simulink model "FormationControl"  (R2021b)
settings: Solver=VariableStepAuto  StartTime=0.0  StopTime=t_sim2  RelTol=1e-3
undefined symbols (not defined in the file or in its folder): d, form
libraries: instrumentlib x1
settings Model: PacingRate=0.100000  Creator=Cinthy  LastModifiedBy=Cinthy

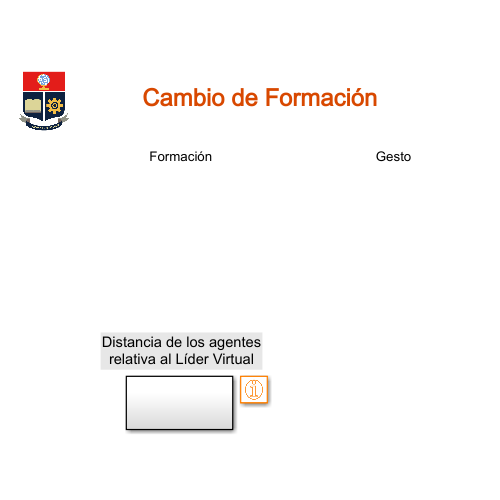
[thumbnail: Simulink's stored preview of the top-level diagram]
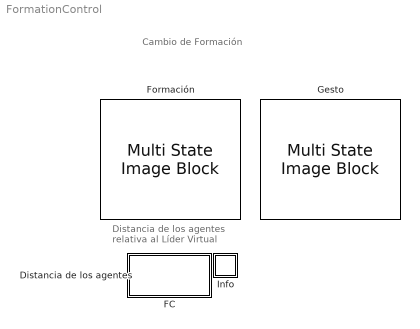
== system FormationControl ==
  note: Distancia de los agentes
      | relativa al Líder Virtual
  note: Cambio de Formación
  Distancia de los agentes : DisplayBlock  LabelPosition=Hide  Format=short  Transparency=1
  FC : Subsystem
  Formación : MultiStateImageBlock  LabelPosition=Hide
  Gesto : MultiStateImageBlock  LabelPosition=Hide
  Info : Subsystem
      mask Display: image('$imagefile'); % Use "Edit Image" on toolstrip to change.

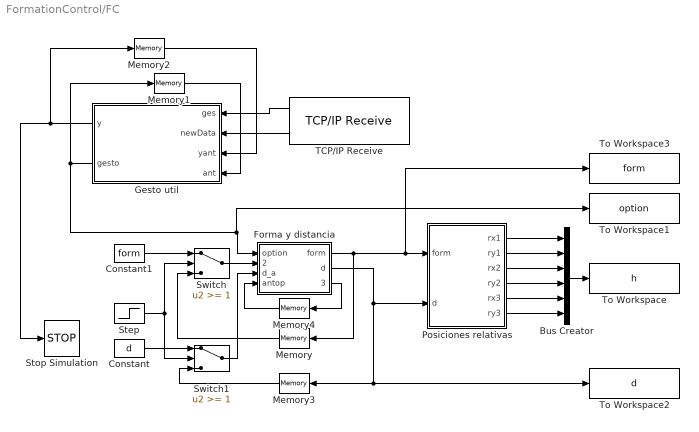
== system FormationControl/FC ==
  Bus Creator : BusCreator  Inputs=6
  Constant : Constant  Value=d
  Constant1 : Constant  Value=form
  Forma y distancia : MATLAB Function  TreatAsAtomicUnit=on
  Gesto util : MATLAB Function  TreatAsAtomicUnit=on
  Memory{,1..4} (5 alike) : Memory
  Posiciones relativas : MATLAB Function  TreatAsAtomicUnit=on
  Step : Step  Time=0.2  Before=1  After=0  SampleTime=0
  Stop Simulation : Stop
  Switch : Switch  Threshold=1
  Switch1 : Switch  Threshold=1
  TCP/IP Receive : instrumentlib/TCP//IP Receive  Host=localhost  Port=3100  DataSize=[ 1, 1 ]  DataType=uint8  ASCIIFormatting=%f  Terminator=LF  CustomTerminator=10  ByteOrder=big-endian  EnableBlockingMode=off  Timeout=10  SampleTime=0.1  SimulateUsing=Interpreted execution
  To Workspace : ToWorkspace  VariableName=h  SampleTime=-1
  To Workspace1 : ToWorkspace  VariableName=option  SampleTime=-1
  To Workspace2 : ToWorkspace  VariableName=d  SampleTime=-1
  To Workspace3 : ToWorkspace  VariableName=form  SampleTime=-1
  wires:
  Forma y distancia/2(d) -> To Workspace2/1, Memory3/1, Posiciones relativas/2(d)
  Switch1/1 -> Forma y distancia/3(d_a)
  Memory/1 -> Switch/3
  Gesto util/2(gesto) -> To Workspace1/1, Forma y distancia/1(option), Memory1/1
  Memory2/1 -> Gesto util/3(yant)
  Step/1 -> Switch/2, Switch1/2
  Posiciones relativas/4(ry2) -> Bus Creator/4
  Forma y distancia/1(form) -> Posiciones relativas/1(form), To Workspace3/1, Memory/1
  Constant1/1 -> Switch/1
  Memory3/1 -> Switch1/3
  Gesto util/1(y) -> Memory2/1, Stop Simulation/1
  Posiciones relativas/1(rx1) -> Bus Creator/1
  Memory1/1 -> Gesto util/4(ant)
  Posiciones relativas/3(rx2) -> Bus Creator/3
  Bus Creator/1 -> To Workspace/1
  TCP/IP Receive/1 -> Gesto util/1(ges)
  TCP/IP Receive/2 -> Gesto util/2(newData)
  Constant/1 -> Switch1/1
  Switch/1 -> Forma y distancia/2(form_a)
  Posiciones relativas/6(ry3) -> Bus Creator/6
  Posiciones relativas/5(rx3) -> Bus Creator/5
  Posiciones relativas/2(ry1) -> Bus Creator/2
  Forma y distancia/3(antges) -> Memory4/1
  Memory4/1 -> Forma y distancia/4(antop)

== system FormationControl/Info ==
  note: Donde d es la distancia que se varía
  note: Distancia relativa en cada eje para cada agente para su posición respecto
      | al Líder Virtual. Ejemplo con la Formación V:

== matlab function FormationControl/FC/Forma y distancia ==
  data: option input; form output; form_a input; d_a input; d output; antop input; antges output
function [form,d,antges] = fcn(option,form_a,d_a,antop)
if option==1&&antop~=1%WaveOut
       form=form_a+1;
       if form==7
           form=6;
       end
       d=d_a;
       antges=1;
elseif option==2&&antop~=2%WaveIn
       form=form_a-1;
       if form==0
          form=1;
       end
       d=d_a;
       antges=2;
elseif option==5&&antop~=5%Pinch
    if d_a==0.5
       d=1.0;
    else
       d=0.5;
    end
    form=form_a;
    antges=5;
else
    form=form_a;
    d=d_a;
    antges=option;
end

== matlab function FormationControl/FC/Gesto util ==
  data: ges input; y output; newData input; gesto output double; yant input; ant input
function [y,gesto]  = stop(ges,newData,yant,ant)
% coder.extrinsic('Simulink.Annotation')
if newData==1
    gesto=double(ges);
    if ges==4||ges==3%open o fist
        y=1;
    else
        y=0;
    end
else
    gesto=ant;
    y=yant;
end

== matlab function FormationControl/FC/Posiciones relativas ==
  data: form input; rx1 output; d input; ry1 output; rx2 output; ry2 output; rx3 output; ry3 output
function [rx1,ry1,rx2,ry2,rx3,ry3] = fcn(form,d)
%rxi,ryi son las posiciones relativas de cada robot respecto al lider vitual
%considerandolo como punto 0,0
if form==1
%         imgform="1columna.png";
%         mssgform="Columna";
        rx1=0; ry1=-d;
        rx2=0; ry2=0;
        rx3=0; ry3=d;
elseif form==2
%         imgform="2fila.png";
%         mssgform="Fila";
        rx1=-d; ry1=0;
        rx2=0; ry2=0;
        rx3=d; ry3=0;
elseif form==3
%         imgform="3V.png";
%         mssgform="Formación V";
        rx1=-d; ry1=d;
        rx2=0; ry2=-d;
        rx3=d; ry3=d;
elseif form==4
%         imgform="4Vinv.png";
%         mssgform="Formación V inversa";
        rx1=-d; ry1=-d;
        rx2=d; ry2=-d;
        rx3=0; ry3=d;
elseif form==5
%         imgform="5L.png";
%         mssgform="Formación L";
        rx1=-d; ry1=-d;
        rx2=d; ry2=-d;
        rx3=-d; ry3=d;
elseif form==6
%         imgform="6Linv.png";
%         mssgform="Formación L inversa";
        rx1=-d; ry1=-d;
        rx2=d; ry2=-d;
        rx3=d; ry3=d;
else
        %         imgform="1columna.png";
%         mssgform="Columna";
        rx1=0; ry1=-d;
        rx2=0; ry2=0;
        rx3=0; ry3=d;
end
